simulink model "Project3"  (R2022a)
settings: Solver=FixedStepAuto  StartTime=0.0  StopTime=inf  FixedStep=0.05  RelTol=1e-3
model workspace (MAT data in the model file):
  SL_ROS_VariableLengthArrays_MaxSizes.CommonInfo.ArrayTruncateAction = 'EmitWarning'
  SL_ROS_VariableLengthArrays_MaxSizes.MsgTypeMap = containers.Map
  SL_ROS_VariableLengthArrays_MaxSizes.MsgTypeMap.serialization.keys = {'sensor_msgs/Image', 'sensor_msgs/LaserScan'}
  SL_ROS_VariableLengthArrays_MaxSizes.MsgTypeMap.serialization.values{1}(1).PropertyName = 'Data'
  SL_ROS_VariableLengthArrays_MaxSizes.MsgTypeMap.serialization.values{1}(1).DataType = 'uint8'
  SL_ROS_VariableLengthArrays_MaxSizes.MsgTypeMap.serialization.values{1}(1).MaxLength = 921600
  SL_ROS_VariableLengthArrays_MaxSizes.MsgTypeMap.serialization.values{1}(2).PropertyName = 'Encoding'
  SL_ROS_VariableLengthArrays_MaxSizes.MsgTypeMap.serialization.values{1}(2).DataType = 'uint8'
  SL_ROS_VariableLengthArrays_MaxSizes.MsgTypeMap.serialization.values{1}(2).MaxLength = 128
  SL_ROS_VariableLengthArrays_MaxSizes.MsgTypeMap.serialization.values{2}(1).PropertyName = 'Intensities'
  SL_ROS_VariableLengthArrays_MaxSizes.MsgTypeMap.serialization.values{2}(1).DataType = 'single'
  SL_ROS_VariableLengthArrays_MaxSizes.MsgTypeMap.serialization.values{2}(1).MaxLength = 360
  SL_ROS_VariableLengthArrays_MaxSizes.MsgTypeMap.serialization.values{2}(2).PropertyName = 'Ranges'
  SL_ROS_VariableLengthArrays_MaxSizes.MsgTypeMap.serialization.values{2}(2).DataType = 'single'
  SL_ROS_VariableLengthArrays_MaxSizes.MsgTypeMap.serialization.values{2}(2).MaxLength = 360
  SL_ROS_VariableLengthArrays_MaxSizes.MsgTypeMap.serialization.uniformity = 0
  SL_ROS_VariableLengthArrays_MaxSizes.MsgTypeMap.serialization.keyType = 'char'
  SL_ROS_VariableLengthArrays_MaxSizes.MsgTypeMap.serialization.valueType = 'any'
undefined symbols (not defined in the file or in its folder): Angular, Linear, Rec, SDTV
libraries: robotlib x7, visionstatistics x2, simulink x2, visionconversions x1
settings Model: Creator=raibuntu  LastModifiedBy=isa
settings OptimizationCC: EnhancedBackFolding=on  PassReuseOutputArgsAs=Individual arguments  ZeroExternalMemoryAtStartup=off  ZeroInternalMemoryAtStartup=off  MaxStackSize=64  OptimizeBlockOrder=speed  DifferentSizesBufferReuse=on  OptimizationCustomize=off  EfficientTunableParamExpr=on
settings DebuggingCC: ParameterTunabilityLossMsg=error
settings HardwareCC: ProdBitPerPointer=32  ProdBitPerSizeT=32  ProdBitPerPtrDiffT=32  ProdLargestAtomicFloat=None  ProdIntDivRoundTo=Undefined  ProdEndianess=Unspecified  ProdWordSize=32  ProdHWDeviceType=Generic->Unspecified (assume 32-bit Generic)
settings ModelReferenceCC: EnableRefExpFcnMdlSchedulingChecks=off
settings SFSimCC: MATLABDynamicMemAlloc=off
settings RTWCC: SystemTargetFile=ert.tlc  HardwareBoard=Robot Operating System (ROS)  TLCOptions="-aInlineSetEventsForThisBaseRateFcn=TLC_FALSE -aSuppressMultiTaskScheduler=TLC_FALSE  -aRateBasedStepFcn=0"  TemplateMakefile=ert_default_tmf  Toolchain=Catkin  TargetLang=C++
settings CodeAppCC: ForceParamTrailComments=on  IgnoreCustomStorageClasses=off  OperatorAnnotations=on  SimulinkDataObjDesc=on  SFDataObjDesc=on  InsertBlockDesc=on

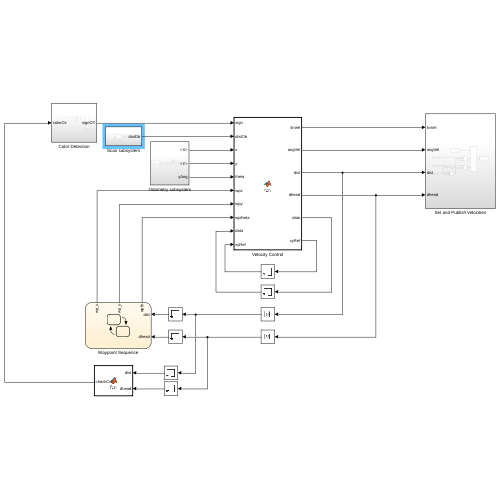
[thumbnail: Simulink's stored preview of the top-level diagram]
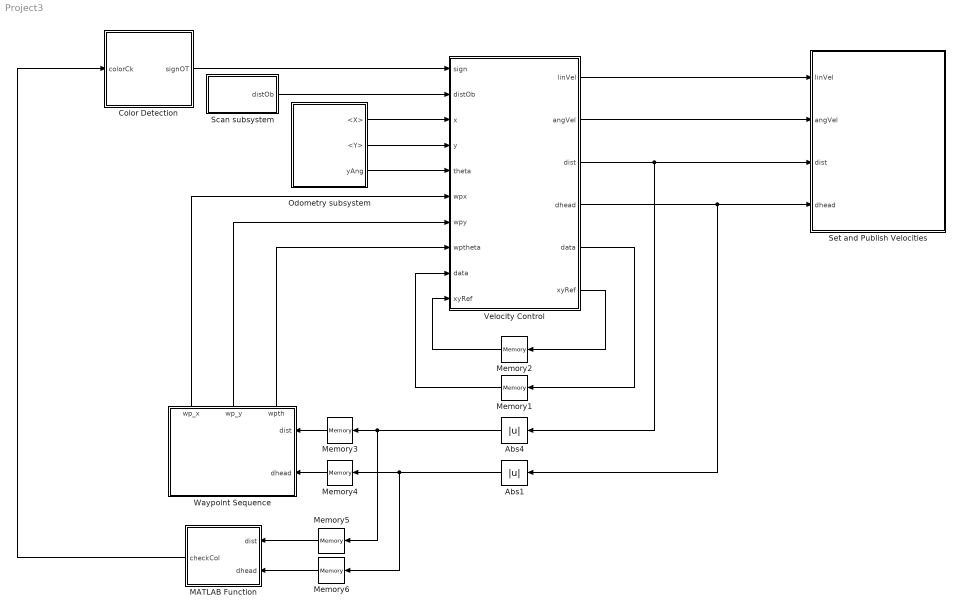
== system Project3 ==
  Abs1 : Abs  SaturateOnIntegerOverflow=off
  Abs4 : Abs  SaturateOnIntegerOverflow=off
  Color Detection : Subsystem
  MATLAB Function : MATLAB Function  TreatAsAtomicUnit=on
  Memory1 : Memory  InitialCondition=[0; 0; 0; 1; 0; 0]
  Memory2 : Memory  InitialCondition=[0 0]
  Memory3 : Memory  InitialCondition=3
  Memory4 : Memory  InitialCondition=1
  Memory5 : Memory
  Memory6 : Memory
  Odometry subsystem : Subsystem
  Scan subsystem : Subsystem
  Set and Publish Velocities : Subsystem
  Velocity Control : MATLAB Function  TreatAsAtomicUnit=on
  Waypoint Sequence : Stateflow chart  TreatAsAtomicUnit=on
      settings: PortSchema="{\"entries\":[{\"content\":{\"sides\":[{\"content\":{\"connectorIds\":[\"In1\",\"In2\"]},\"type\":\"ConnectorPlacement.EquallySpacedRectSide\",\"uuid\":\"3c0b8c44-7056-474e-88d4-c274adb67b29\"},{\"content\":{\"connectorIds\":[],\"side\":\"RIGHT\"},\"type\":\"ConnectorPlacement.EquallySpacedRectSide\",\"uuid\":\"34274f05-3395-441e-bdde-745717c201d9\"},{\"content\":{\"connectorIds\":[\"Out1\",\"Out3\",\"Out2\"],\"side\":\"TOP\"},\"type\":\"ConnectorPlacement.EquallySpacedRectSide\",\"uuid\":\"2ace7ecf-149b-4880-9112-b92e722c30ce\"}]},\"type\":\"ConnectorPlacement.EquallySpacedConnector\",\"uuid\":\"13a72b12-83d7-40ce-b575-face567932a9\"}],\"packageUris\":[\"http://schema.mathworks.com/mf0/Connector/R2020b\"],\"version\":\"1.0\"}"
  wires:
  Waypoint Sequence/1(wpth) -> Velocity Control/8(wptheta)
  Odometry subsystem/3(yAng) -> Velocity Control/5(theta)
  Memory1/1 -> Velocity Control/9("data ")
  Odometry subsystem/1(<X>) -> Velocity Control/3(x)
  Velocity Control/6(xyRef) -> Memory2/1
  Memory2/1 -> Velocity Control/10("xyRef ")
  Odometry subsystem/2(<Y>) -> Velocity Control/4(y)
  Velocity Control/3(dist) -> Abs4/1, Set and Publish Velocities/3(dist)
  Velocity Control/5(data) -> Memory1/1
  Memory3/1 -> Waypoint Sequence/1(dist)
  Waypoint Sequence/3(wp_y) -> Velocity Control/7(wpy)
  Waypoint Sequence/2(wp_x) -> Velocity Control/6(wpx)
  Scan subsystem/1(distOb) -> Velocity Control/2(distOb)
  Abs1/1 -> Memory6/1, Memory4/1
  Abs4/1 -> Memory5/1, Memory3/1
  Memory4/1 -> Waypoint Sequence/2(dhead)
  Color Detection/1(signOT) -> Velocity Control/1(sign)
  Memory5/1 -> MATLAB Function/1(dist)
  Memory6/1 -> MATLAB Function/2(dhead)
  MATLAB Function/1(checkCol) -> Color Detection/1(colorCk)
  Velocity Control/4(dhead) -> Abs1/1, Set and Publish Velocities/4(dhead)
  Velocity Control/1(linVel) -> Set and Publish Velocities/1(linVel)
  Velocity Control/2(angVel) -> Set and Publish Velocities/2(angVel)

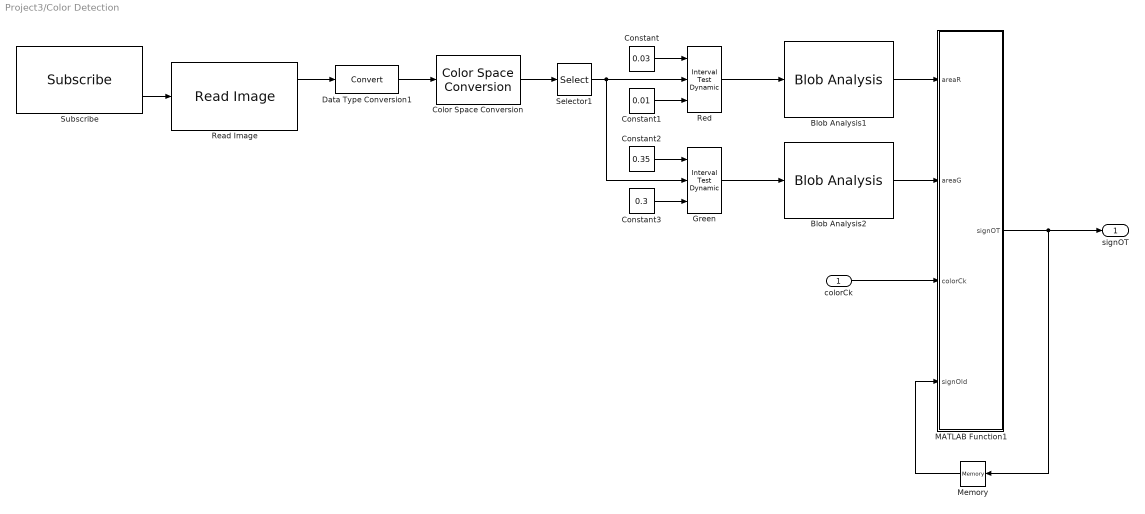
== system Project3/Color Detection ==
  colorCk : Inport
  Blob Analysis1 : visionstatistics/Blob Analysis  Tag=vipblks_row_conv  area=on  centroid=off  bBox=off  majorAxis=off  minorAxis=off  angle=off  eccentricity=off  equivDiameterSq=off  extent=off  perimeter=off  outDT=double  conn=8  isLabel=off  maxBlobs=6  warnIfNumBlobsExceeded=on  isCount=off  useMinArea=off  minArea=0  useMaxArea=off  maxArea=intmax('uint32')  excludeBorderBlob=off  isOutVarDim=off  isFill=on  fillValues=-1  roundingMode=Floor  overflowMode=off  prodOutputMode=Binary point scaling  prodOutputWordLength=32  prodOutputFracLength=16  accumMode=Binary point scaling  accumWordLength=32  accumFracLength=0  outputMode=Binary point scaling  outputWordLength=32  outputFracLength=16  firstCoeffMode=Binary point scaling  firstCoeffWordLength=16  firstCoeffFracLength=14  secondCoeffMode=Binary point scaling  secondCoeffWordLength=32  secondCoeffFracLength=16
  Blob Analysis2 : visionstatistics/Blob Analysis  Tag=vipblks_row_conv  area=on  centroid=off  bBox=off  majorAxis=off  minorAxis=off  angle=off  eccentricity=off  equivDiameterSq=off  extent=off  perimeter=off  outDT=double  conn=8  isLabel=off  maxBlobs=6  warnIfNumBlobsExceeded=on  isCount=off  useMinArea=off  minArea=0  useMaxArea=off  maxArea=intmax('uint32')  excludeBorderBlob=off  isOutVarDim=off  isFill=on  fillValues=-1  roundingMode=Floor  overflowMode=off  prodOutputMode=Binary point scaling  prodOutputWordLength=32  prodOutputFracLength=16  accumMode=Binary point scaling  accumWordLength=32  accumFracLength=0  outputMode=Binary point scaling  outputWordLength=32  outputFracLength=16  firstCoeffMode=Binary point scaling  firstCoeffWordLength=16  firstCoeffFracLength=14  secondCoeffMode=Binary point scaling  secondCoeffWordLength=32  secondCoeffFracLength=16
  Color Space Conversion : visionconversions/Color Space  Conversion  conversion=Obsolete  conversionActive=R'G'B' to HSV  wp_str=D65  rec=Rec. 601 (SDTV)  sys=1125/60/2:1  imagePorts=One multidimensional signal
  Constant : Constant  Value=0.03
  Constant1 : Constant  Value=0.01
  Constant2 : Constant  Value=0.35
  Constant3 : Constant  Value=0.3
  Data Type Conversion1 : DataTypeConversion  SaturateOnIntegerOverflow=off  RndMeth=Floor
  Green : simulink/Logic and Bit Operations/Interval Test Dynamic  IntervalClosedRight=on  IntervalClosedLeft=on  OutDataTypeStr=boolean
      settings: SourceProductBaseCode=SL
  MATLAB Function1 : MATLAB Function  TreatAsAtomicUnit=on
  Memory : Memory
  Read Image : robotlib/Read Image  MaximumImageSize=[480, 640]  ImageEncoding=rgb8  ShowAlphaOutput=off  ShowErrorCodeOutput=on  VariableSizeOutputs=off
      settings: SourceProductBaseCode=RR
  Red : simulink/Logic and Bit Operations/Interval Test Dynamic  IntervalClosedRight=on  IntervalClosedLeft=on  OutDataTypeStr=boolean
      settings: SourceProductBaseCode=SL
  Selector1 : Selector  NumberOfDimensions=3  InputPortWidth=3  IndexOptions=Index vector (dialog),Index vector (dialog),Index vector (dialog)  Indices=[1:480],[1:640],1  OutputSizes=1,1,1
  Subscribe : robotlib/Subscribe  topicSource=Select from ROS network  topic=/camera/rgb/image_raw  messageType=sensor_msgs/Image  SampleTime=-1  legacyBusStruct=off  messageQueueLength=1
  signOT : Outport
  wires:
  Color Space Conversion/1 -> Selector1/1
  Constant/1 -> Red/1
  Blob Analysis1/1 -> MATLAB Function1/1(areaR)
  Subscribe/2 -> Read Image/1
  Constant2/1 -> Green/1
  Selector1/1 -> Red/2, Green/2
  Read Image/1 -> Data Type Conversion1/1
  Blob Analysis2/1 -> MATLAB Function1/2(areaG)
  Constant3/1 -> Green/3
  Red/1 -> Blob Analysis1/1
  Constant1/1 -> Red/3
  Green/1 -> Blob Analysis2/1
  Data Type Conversion1/1 -> Color Space Conversion/1
  MATLAB Function1/1(signOT) -> signOT/1, Memory/1
  Memory/1 -> MATLAB Function1/4(signOld)
  colorCk/1 -> MATLAB Function1/3(colorCk)

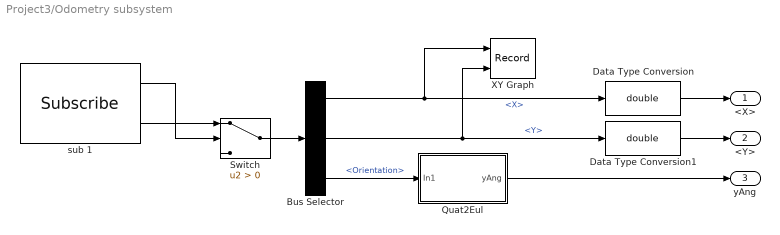
== system Project3/Odometry subsystem ==
  Bus Selector : BusSelector  OutputSignals=Pose.Pose.Position.X,Pose.Pose.Position.Y,Pose.Pose.Orientation
  Data Type Conversion : DataTypeConversion  OutDataTypeStr=double  SaturateOnIntegerOverflow=off  RndMeth=Floor
  Data Type Conversion1 : DataTypeConversion  OutDataTypeStr=double  SaturateOnIntegerOverflow=off  RndMeth=Floor
  Quat2Eul : Subsystem
  Switch : Switch  Criteria=u2 > Threshold  SaturateOnIntegerOverflow=off  InputSameDT=off
  XY Graph : Record  FileSettingsInternal="{\"entries\":[{\"content\":{\"excelSettings\":{\"content\":{},\"type\":\"Streamout.ExcelSettings\"}},\"type\":\"Streamout.FileSettingStorage\",\"uuid\":\"fa819d97-8a01-4fd8-bb4c-c4b8b7be5a71\"}],\"packageUris\":[\"http://schema.mathworks.com/mf0/streamout_blocks/R2020a\"],\"version\":\"1.0\"}"  Layout=[1 1]  SignalsInternal="{\"entries\":[{\"content\":{\"signals\":[{\"content\":{\"blockPath\":[\"Project3/Odometry subsystem/XY Graph\"],\"channel\":[],\"dimensions\":[1],\"domain\":\"Project3/Odometry subsystem/XY Graph\",\"lineColor\":\"#a2142f\",\"plots\":[1],\"port\":1,\"sid\":[],\"signalID\":36,\"signalName\":\"<X>\"},\"type\":\"RecordBlkView.Signal\",\"uuid\":\"443fe2d9-428c-494c-93ec-7669d18c38f7\"},{\"content\":{\"blockPath\":[\"Project3/Odometry subsystem/XY Graph\"],\"channel\":[],\"dimensions\":[1],\"domain\":\"Project3/Odometry subsystem/XY Graph\",\"lineColor\":\"#139fff\",\"plots\":[1],\"port\":2,\"sid\":[],\"signalID\":39,\"signalName\":\"<Y>\"},\"type\":\"RecordBlkView.Signal\",\"uuid\":\"b3429a7f-796e-4852-a97b-3fea679ec065\"}]},\"type\":\"RecordBlkView.InputSignals\",\"uuid\":\"bfd1a354-9c90-4848-a290-45dfe56bcabc\"}],\"packageUris\":[\"http://schema.mathworks.com/mf0/streamout_blocks/R2020a\"],\"version\":\"1.0\"}"  VisualizationBindings="{\"xyplotplugin\":{\"info\":[{\"series\":[{\"bindingParametersList\":[{\"parameter\":\"X-Axis\",\"signalID\":36,\"signalName\":\"<X>\"},{\"parameter\":\"Y-Axis\",\"signalID\":39,\"signalName\":\"<Y>\"}],\"seriesID\":3556}],\"subplotID\":1}]}}"  CompatibilityTag=XY  st=-1
  sub 1 : robotlib/Subscribe  topicSource=Select from ROS network  topic=/odom  messageType=nav_msgs/Odometry  SampleTime=-1  legacyBusStruct=off  messageQueueLength=51
  <X> : Outport
  <Y> : Outport  Port=2
  yAng : Outport  Port=3
  wires:
  Bus Selector/3 -> Quat2Eul/1(In1)  "<Orientation>"
  Switch/1 -> Bus Selector/1
  Bus Selector/1 -> XY Graph/1, Data Type Conversion/1  "<X>"
  sub 1/1 -> Switch/2
  sub 1/2 -> Switch/1
  Quat2Eul/1(yAng) -> yAng/1
  Bus Selector/2 -> XY Graph/2, Data Type Conversion1/1  "<Y>"
  Data Type Conversion/1 -> <X>/1
  Data Type Conversion1/1 -> <Y>/1

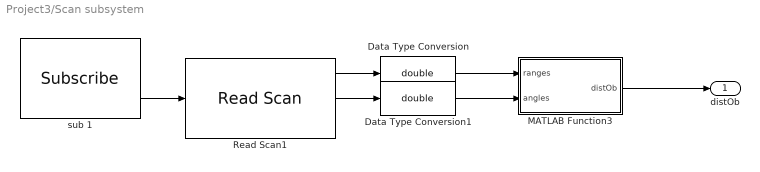
== system Project3/Scan subsystem ==
  Data Type Conversion : DataTypeConversion  OutDataTypeStr=double  SaturateOnIntegerOverflow=off  RndMeth=Floor
  Data Type Conversion1 : DataTypeConversion  OutDataTypeStr=double  SaturateOnIntegerOverflow=off  RndMeth=Floor
  MATLAB Function3 : MATLAB Function  TreatAsAtomicUnit=on
  Read Scan1 : robotlib/Read Scan  MaximumArrayLength=360  ShowAnglesOutput=on  ShowIntensityOutput=off  ShowErrorCodeOutput=on  VariableSizeOutputs=off
      settings: SourceProductBaseCode=RR
  sub 1 : robotlib/Subscribe  topicSource=Select from ROS network  topic=/scan  messageType=sensor_msgs/LaserScan  SampleTime=-1  legacyBusStruct=off  messageQueueLength=51
  distOb : Outport
  wires:
  sub 1/2 -> Read Scan1/1
  Read Scan1/1 -> Data Type Conversion/1
  Read Scan1/2 -> Data Type Conversion1/1
  MATLAB Function3/1(distOb) -> distOb/1
  Data Type Conversion/1 -> MATLAB Function3/1(ranges)
  Data Type Conversion1/1 -> MATLAB Function3/2(angles)

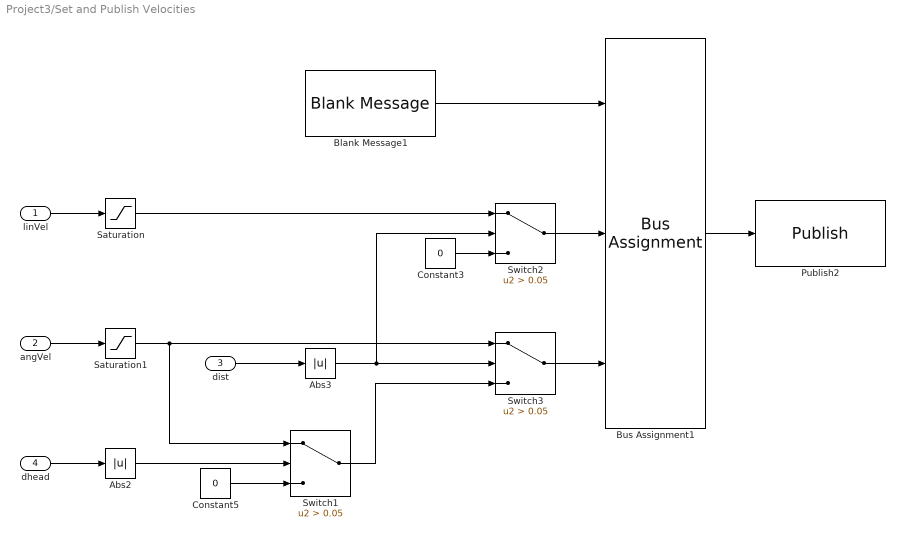
== system Project3/Set and Publish Velocities ==
  linVel : Inport
  angVel : Inport  Port=2
  dist : Inport  Port=3
  dhead : Inport  Port=4
  Abs2 : Abs  SaturateOnIntegerOverflow=off
  Abs3 : Abs  SaturateOnIntegerOverflow=off
  Blank Message1 : robotlib/Blank Message  messageClass=Message  entityType=geometry_msgs/Twist  messageType=geometry_msgs/Twist  SampleTime=inf  legacyBusStruct=off
  Bus Assignment1 : BusAssignment  DialogController=Simulink.DDGSource_BusAssignment  AssignedSignals=Linear.X,Angular.Z
  Constant3 : Constant  Value=0
  Constant5 : Constant  Value=0
  Publish2 : robotlib/Publish  topicSource=Select from ROS network  topic=/cmd_vel  messageType=geometry_msgs/Twist  legacyBusStruct=off  messageQueueLength=105
  Saturation : Saturate  UpperLimit=0.1  LowerLimit=-0.1
  Saturation1 : Saturate  UpperLimit=0.4  LowerLimit=-0.4
  Switch1 : Switch  Criteria=u2 > Threshold  Threshold=0.05  SaturateOnIntegerOverflow=off  InputSameDT=off
  Switch2 : Switch  Criteria=u2 > Threshold  Threshold=0.05  SaturateOnIntegerOverflow=off  InputSameDT=off
  Switch3 : Switch  Criteria=u2 > Threshold  Threshold=0.05  SaturateOnIntegerOverflow=off  InputSameDT=off
  wires:
  Switch2/1 -> Bus Assignment1/2
  Saturation1/1 -> Switch3/1, Switch1/1
  linVel/1 -> Saturation/1
  Switch1/1 -> Switch3/3
  Abs2/1 -> Switch1/2
  Constant3/1 -> Switch2/3
  Constant5/1 -> Switch1/3
  Abs3/1 -> Switch3/2, Switch2/2
  dist/1 -> Abs3/1
  Switch3/1 -> Bus Assignment1/3
  dhead/1 -> Abs2/1
  Saturation/1 -> Switch2/1
  Bus Assignment1/1 -> Publish2/1
  Blank Message1/1 -> Bus Assignment1/1
  angVel/1 -> Saturation1/1

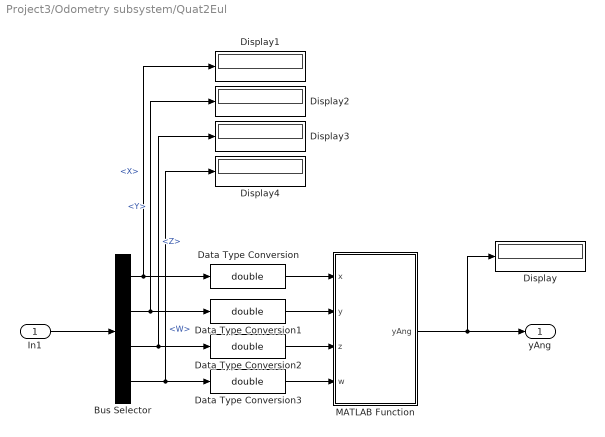
== system Project3/Odometry subsystem/Quat2Eul ==
  In1 : Inport
  Bus Selector : BusSelector  OutputSignals=X,Y,Z,W
  Data Type Conversion{,1..3} (4 alike) : DataTypeConversion  OutDataTypeStr=double  SaturateOnIntegerOverflow=off  RndMeth=Floor
  Display{,1..4} (5 alike) : Display
  MATLAB Function : MATLAB Function  TreatAsAtomicUnit=on
  yAng : Outport
  wires:
  In1/1 -> Bus Selector/1
  MATLAB Function/1(yAng) -> Display/1, yAng/1
  Bus Selector/2 -> Display2/1, Data Type Conversion1/1  "<Y>"
  Bus Selector/1 -> Data Type Conversion/1, Display1/1  "<X>"
  Bus Selector/3 -> Display3/1, Data Type Conversion2/1  "<Z>"
  Bus Selector/4 -> Display4/1, Data Type Conversion3/1  "<W>"
  Data Type Conversion/1 -> MATLAB Function/1(x)
  Data Type Conversion1/1 -> MATLAB Function/2(y)
  Data Type Conversion2/1 -> MATLAB Function/3(z)
  Data Type Conversion3/1 -> MATLAB Function/4(w)

== matlab function Project3/Odometry subsystem/Quat2Eul/MATLAB Function ==
  data: x input; yAng output; y input; z input; w input
function yAng = conversAngle(x,y,z,w)
eulAngle = quat2eul([w,x,y,z]);
yAng = eulAngle(1);
check = isnan(yAng);
if check == 1
    yAng = 0;
end
end

== matlab function Project3/Color Detection/MATLAB Function1 ==
  data: areaR input; areaG input; colorCk input; signOT output; signOld input
function signOT  = fcn(areaR,areaG,colorCk,signOld)

[maxAreaG,iG] = max(areaG);
[maxAreaR,iR] = max(areaR);

if colorCk == 1
    if ~isempty(iG) && ~isempty(iR) 
        if maxAreaR > maxAreaG
            signOT =-1;
        elseif maxAreaG > maxAreaR
            signOT = 1;
        else
            signOT = signOld;
        end
    else 
        signOT = signOld;
    end
else
    signOT = signOld;
end

== matlab function Project3/MATLAB Function ==
  data: dist input; checkCol output; dhead input
function checkCol = fcn(dist,dhead)
if dist<0.05 && dhead<0.05
    checkCol = 1;
else
    checkCol = 0;
end
end

== stateflow chart Project3/Waypoint Sequence ==
  settings: executeAtInitialization=1
  state Waypoint1
    entry: wp_x=4; wp_y=0; wpth = pi/2;
  state Waypoint2
    entry: wp_x=4; wp_y=4; wpth = pi/2;
  state Waypoint3
    entry: wp_x=4; wp_y=8; wpth = 0;
  state Waypoint4
    entry: wp_x=8; wp_y=8; wpth =3*pi/2;
  state Waypoint5
    entry: wp_x=8; wp_y=4; wpth = 3*pi/2;
  state Waypoint6
    entry: wp_x=8; wp_y=0; wpth = 3*pi/2;
  (default) -> Waypoint1
  Waypoint1 -> Waypoint2 : [dist<0.05 & dhead <0.05]
  Waypoint2 -> Waypoint3 : [dist<0.05 & dhead <0.05]
  Waypoint3 -> Waypoint4 : [dist<0.05 & dhead <0.05]
  Waypoint4 -> Waypoint5 : [dist<0.05 & dhead <0.05]
  Waypoint5 -> Waypoint6 : [dist<0.05 & dhead <0.05]
  Waypoint6 -> Waypoint6 : [dist<0.05 & dhead <0.05]
  data: wpth output; dist input double; wp_x output double; wp_y output double; dhead input

== matlab function Project3/Scan subsystem/MATLAB Function3 ==
  data: ranges input; angles input; distOb output
function distOb  = fcn(ranges,angles)
if any(ranges>0)
    xOb     = ranges.*cos(angles);
    yOb     = ranges.*sin(angles);
    % only return finite values
    xObVal     = xOb(isfinite(xOb));
    yObVal     = yOb(isfinite(yOb));
    distOb  = min(sqrt(xObVal.^2 + yObVal.^2));
else
    distOb = 0;
end

== matlab function Project3/Velocity Control ==
  data: sign input; distOb input; linVel output; x input; y input; theta input; wpx input; wpy input; wptheta input; data input; xyRef input; angVel output; dist output; dhead output; data output; xyRef output
function [linVel,angVel,dist,dhead,data,xyRef] = fcn(sign,distOb,x,y,theta,wpx,wpy,wptheta,data,xyRef)
check   = data(1);
checkP  = data(2);
R       = data(3);
distOT  = data(4);
distRef = data(5);
theta0  = data(6);

dist    = sqrt((x - wpx)^2 + (y - wpy)^2);
course  = atan2(wpy - y,wpx - x);

kpv     = 0.07;
kpw     = 0.07;

if distOb < 1 && distOb > 0
     distOT = distOb;
end

if distOT < 1 && distRef <= 1.3*R
    if checkP == 0
        theta0 = theta;
        checkP = 1;
    end
    if check == 0 
        ang     = -sign*pi/2 + theta0;
        perp    = abs(ang - theta);
        if abs(perp) <= 0.03
            linVel      = 0;
            angVel      = 0;
            xyRef(1)    = x;
            xyRef(2)    = y;
            R           = distOT + 0.1; 
            distRef     = sqrt((x - xyRef(1))^2 + (y - xyRef(2))^2);
            check       = 1;
        else 
            linVel  = 0;
            angVel  = -sign*kpw*perp;
            check   = 0;
        end
    else
        angVel  = sign*0.06;
        linVel  = abs(angVel)*R;
        distRef = sqrt((x - xyRef(1))^2 + (y - xyRef(2))^2);
        check   = 1;
    end
    dhead = 1;
else
    if dist <= 0.05 
        if theta < 0
            wptheta = wptheta - 2*pi;
        end
        dhead = wptheta - theta;
        check = 0;
        checkP = 0;
        distRef = 0;
        distOT = 1;
        theta0 = 0;
    else
        dhead0 = course - theta;
        if dhead0 < -pi
            dhead = dhead0 + 2*pi;
        elseif dhead0 > pi
            dhead = dhead0 - 2*pi;
        else
            dhead = dhead0;
        end
    end
    linVel  = kpv*dist;
    angVel  = kpw*dhead;
end

data(1) = check;
data(2) = checkP;
data(3) = R;
data(4) = distOT;
data(5) = distRef;
data(6) = theta0;
end
